simulink model "prach_shortFormat_fftShift_chanfix"  (R2022a)
settings: Solver=FixedStepDiscrete  StartTime=0.0  StopTime=prach_short.SimulationTime  FixedStep=1  RelTol=1e-3  EnableMultiTasking=on
PreLoadFcn:
  | warning off Simulink:Commands:SetParamLinkChangeWarn
  | warning off Simulink:Commands:LoadMdlParameterizedLink
  | warning off Simulink:SL_SetParamLinkChangeWarn
  | warning off Simulink:SL_LoadMdlParameterizedLink
  | setup_prach_shortFormat_fftShift;
InitFcn:
  | setup_prach_shortFormat_fftShift;
StopFcn:
  | figure;
  | subplot(3,1,1);
  | plot(real(X(:,1))/max(real(X(:,1))),'b');
  | hold on;
  | plot(imag(X(:,1))/max(real(X(:,1))),'r');
  | title('Raw FFT output, matlab reference');
  | subplot(3,1,2);
  | plot(real(PrachOut_DSPBA(1:Nfft))/max(real(PrachOut_DSPBA(1:Nfft))), 'k');
  | hold on;
  | plot(imag(PrachOut_DSPBA(1:Nfft))/max(imag(PrachOut_DSPBA(1:Nfft))), 'm');
  | title('Raw FFT output, DSP Builder');
  | subplot(3,1,3);
  | plot(real(X(:,1))/max(real(X(:,1)))-real(PrachOut_DSPBA(1:Nfft))/max(real(PrachOut_DSPBA(1:Nfft))), 'g');
  | hold on;
  | plot(imag(X(:,1))/max(real(X(:,1)))-imag(PrachOut_DSPBA(1:Nfft))/max(imag(PrachOut_DSPBA(1:Nfft))), 'c');
  | title('Difference');
  | 
  | figure;
  | subplot(2,1,1);
  | plot(real(prach_output(:,1))/max(real(prach_output(:,1))),'b');
  | hold on;
  | plot(imag(prach_output(:,1))/max(real(prach_output(:,1))),'r');
  | title('PRACH output, matlab, normalized ');
  | subplot(2,1,2);
  | for i=1:139
  |     PrachOut139reordered_DSPBA(1+PrachIdxOut139_DSPBA(i)) = PrachOut139_DSPBA(i);
  | end;
  | plot(real(PrachOut139reordered_DSPBA)/max(real(PrachOut139reordered_DSPBA)), 'k');
  | hold on;
  | plot(imag(PrachOut139reordered_DSPBA)/max(imag(PrachOut139reordered_DSPBA)), 'm');
  | title('PRACH output, DSP Builder, normalized');
values from neighbouring files (symbols this model uses):
  ConfigTable = [16 1 9,20,20,20,20,20,20,20,20,20 0 2 6 2 4 ... (first row only)    [ConfigIndexTable.m]
  NTxAnts = 4    [setup_prach_shortFormat.m]    (also in setup_prach_shortFormat_fftShift.m)
undefined symbols (not defined in the file or in its folder): AdvDSPBChannelOutDisplay, AdvDSPBDMemDisplay, BW, ControlDecode, display, dpoly, dspba, dspba_ChannelInVis, dspba_ChannelOutVis, dspba_internal_get_channel_ports, evalAionMaskParam, latency, PRACH_CC, PRACH_regs, prach_short, PrachLib, PrachLib_FFTshift, primtype, RemoveCP, Stream2BlockConv, UseDontCare, value, waveconfig
libraries: DSPBAPrim x326, DSPBAControl x10, DSPBAModelBus x7, DSPBABase x5, DSPBAUtilities x5, simulink x2, DSPBAVectorUtil x1, DspbAdvFftLibrary x1
(part 1 of 5)
Description:
  | This design Implements a PRACH detection for short format for TDD configurations.
settings Model: Creator=lrigby  LastModifiedBy=5g
settings SolverCC: AlgebraicLoopSolver=TrustRegion
settings DataIOCC: LimitDataPoints=on  SaveFormat=StructureWithTime  SignalLoggingSaveFormat=ModelDataLogs  ReturnWorkspaceOutputs=off
settings OptimizationCC: ExpressionDepthLimit=2147483647  InitFltsAndDblsToZero=on  LifeSpan=inf
settings DebuggingCC: SaveWithParameterizedLinksMsg=none  UnderspecifiedInitializationDetection=Classic  MergeDetectMultiDrivingBlocksExec=none  SignalResolutionControl=TryResolveAllWithWarning  SolverPrmCheckMsg=warning  ParameterPrecisionLossMsg=none  UnconnectedInputMsg=warning  UnconnectedOutputMsg=warning  UnconnectedLineMsg=warning  StateNameClashWarn=warning  SFUnexpectedBacktrackingDiag=warning  SFNoUnconditionalDefaultTransitionDiag=warning  SFExecutionAtInitializationDiag=none  ArithmeticOperatorsInVariantConditions=warning
settings HardwareCC: ProdBitPerPointer=32  ProdBitPerSizeT=32  ProdBitPerPtrDiffT=32  ProdLargestAtomicFloat=None  ProdIntDivRoundTo=Undefined  ProdEndianess=Unspecified  ProdWordSize=32  ProdHWDeviceType=ASIC/FPGA  TargetBitPerLong=64  TargetBitPerPointer=64  TargetBitPerSizeT=64  TargetBitPerPtrDiffT=64  TargetLongLongMode=on  TargetIntDivRoundTo=Zero  TargetEndianess=LittleEndian  TargetWordSize=64  TargetHWDeviceType=MATLAB Host  ProdEqTarget=off
settings ModelReferenceCC: PropagateSignalLabelsOutOfModel=off
settings SFSimCC: SimUseLocalCustomCode=off  SimParseCustomCode=off  CustomCodeUndefinedFunction=UseInterfaceOnly
settings RTWCC: RTWUseLocalCustomCode=off  DLArmComputeVersion=19.05
settings CodeAppCC: StateflowObjectComments=on
settings GRTTargetCC: TargetFcnLib=ansi_tfl_tmw.mat  TargetLangStandard=C89/C90 (ANSI)  CombineOutputUpdateFcns=off  GRTInterface=on
settings ConfigComp: CovMetricSettings=dw  CovSaveCumulativeToWorkspaceVar=on  CovSaveSingleToWorkspaceVar=on  CovExternalEMLEnable=off  CovSFcnEnable=off

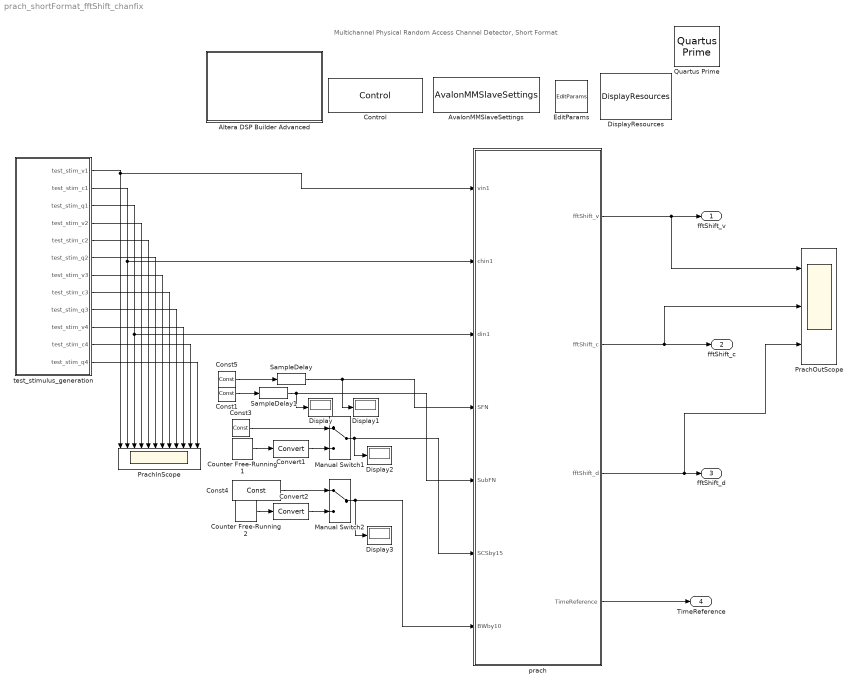
== system prach_shortFormat_fftShift_chanfix ==
  note: Multichannel Physical Random
      | Access Channel Detector, Short Format
  Altera DSP Builder Advanced : Subsystem  mask(DSP Builder Advanced Blockset Ignored Block){}
      settings: OpenFcn=web('http://www.altera.com', '-new');
      mask Display: image(imread('alteralogo.tif'));
  AvalonMMSlaveSettings : DSPBABase/AvalonMMSlaveSettings
  Const1 : DSPBAPrim/Const  primtype=const  nInputs=0  nOutputs=1  omode=Specify via dialog  otype=uint(8)  scale=2^-0  rndmethod=Unbiased  factor=1  satmethod=Symmetric  shift_vec=[0 1 2 -1]  value=SubF  inPortNames=['+'; '+';]  outPortNames=[' ']  dspbaimage=dspba_prim.svg  text=fprintf('%s', num2str(value));  style=Optimised  visibilities=8 + 1024  floatPrecision=float32_m23  warnSaturation=on  version=20211007  SampleTime=inf
  Const3 : DSPBAPrim/Const  primtype=const  nInputs=0  nOutputs=1  omode=Specify via dialog  otype=uint(2)  scale=1  rndmethod=Unbiased  factor=1  satmethod=Symmetric  shift_vec=[0 1 2 -1]  value=floor(waveconfig.PRACH.Config.SubcarrierSpacing/15)  inPortNames=['+'; '+';]  outPortNames=[' ']  dspbaimage=dspba_prim.svg  text=fprintf('%s', num2str(value));  style=Optimised  visibilities=8 + 1024  floatPrecision=float32_m23  warnSaturation=on  version=20211007  SampleTime=inf
  Const4 : DSPBAPrim/Const  primtype=const  nInputs=0  nOutputs=1  omode=Specify via dialog  otype=uint(4)  scale=1  rndmethod=Unbiased  factor=1  satmethod=Symmetric  shift_vec=[0 1 2 -1]  value=floor(BW/10)  inPortNames=['+'; '+';]  outPortNames=[' ']  dspbaimage=dspba_prim.svg  text=fprintf('%s', num2str(value));  style=Optimised  visibilities=8 + 1024  floatPrecision=float32_m23  warnSaturation=on  version=20211007  SampleTime=inf
  Const5 : DSPBAPrim/Const  primtype=const  nInputs=0  nOutputs=1  omode=Specify via dialog  otype=uint(12)  scale=2^-0  rndmethod=Unbiased  factor=1  satmethod=Symmetric  shift_vec=[0 1 2 -1]  value=SFN  inPortNames=['+'; '+';]  outPortNames=[' ']  dspbaimage=dspba_prim.svg  text=fprintf('%s', num2str(value));  style=Optimised  visibilities=8 + 1024  floatPrecision=float32_m23  warnSaturation=on  version=20211007  SampleTime=inf
  Control : DSPBABase/Control  generate=on  language=VHDL  destination=./rtl  make_full_path=off  path_is_relative=on  autotestbench=on  signaldepth=2  coveragetestbench=off  logs=off  spacewidth=2  spacenum=1  addrwidth=10  datawidth=16  dataendian=Big Endian  hierarchicalnames=on  ramThresholdBits=-1  distRamThresholdBits=-1  mlabThresholdBits=-1  hardMultiplierThresholdLuts=-1  version=20090407  errorOnChanMismatch=1  errorOnGPIOMismatch=0  importModelsimResults=0  cycleAccurate=off  reinterpretCastMult=off  paramFile=prach_shortFormat_fftShift_params.xml
  Convert1 : DSPBAPrim/Convert  primtype=convert  nInputs=1  nOutputs=1  omode=Specify via dialog  otype=uint(2)  scale=1  rndmethod=Biased  factor=1  satmethod=None  shift_vec=[0 1 2 -1]  value=round([0:255]/17)  inPortNames=[' '; ' ';]  outPortNames=[' '; 'c']  dspbaimage=dspba_prim_wide.svg  text=fprintf('convert');  style=Optimised  visibilities=8+64+256+2^17  clipdetect=off  floatPrecision=float32_m23  advOptions=[]  version=20211007
  Convert2 : DSPBAPrim/Convert  primtype=convert  nInputs=1  nOutputs=1  omode=Specify via dialog  otype=uint(8)  scale=1  rndmethod=Biased  factor=1  satmethod=None  shift_vec=[0 1 2 -1]  value=round([0:255]/17)  inPortNames=[' '; ' ';]  outPortNames=[' '; 'c']  dspbaimage=dspba_prim_wide.svg  text=fprintf('convert');  style=Optimised  visibilities=8+64+256+2^17  clipdetect=off  floatPrecision=float32_m23  advOptions=[]  version=20211007
  Counter Free-Running1 : simulink/Sources/Counter Free-Running  NumBits=2  tsamp=-1
  Counter Free-Running2 : simulink/Sources/Counter Free-Running  NumBits=4  tsamp=-1
  Display{,1..3} (4 alike) : Display
  DisplayResources : DSPBAUtilities/DisplayResources  mults=0  luts=0  memorybits=0
  EditParams : DSPBABase/EditParams  version=20090407
  Manual Switch1 : ManualSwitch
  Manual Switch2 : ManualSwitch
  PrachInScope : Scope  NumInputPorts=12
  PrachOutScope : Scope  NumInputPorts=3
  Quartus Prime : DSPBABase/Quartus Prime  version=20090407
  SampleDelay : DSPBAPrim/SampleDelay  primtype=sampdelay  nInputs=1  nOutputs=1  omode=Inherit via internal rule  otype=sfix(16)  scale=2^-15  rndmethod=Unbiased  factor=1  satmethod=Symmetric  shift_vec=[0 1 2 -1]  floatPrecision=float32_m23  value=0  inPortNames=[' '; ' ';]  outPortNames=[' ']  dspbaimage=dspba_prim.svg  text=dpoly(1, eye(1,value+1), 'z')  style=Optimised  visibilities=8 + 1024 + 2^17 + 2^18  flexible=off  slackgroup=0  augmented=0  version=20211007  advOptions=[]
  SampleDelay1 : DSPBAPrim/SampleDelay  primtype=sampdelay  nInputs=1  nOutputs=1  omode=Inherit via internal rule  otype=sfix(16)  scale=2^-15  rndmethod=Unbiased  factor=1  satmethod=Symmetric  shift_vec=[0 1 2 -1]  floatPrecision=float32_m23  value=0  inPortNames=[' '; ' ';]  outPortNames=[' ']  dspbaimage=dspba_prim.svg  text=dpoly(1, eye(1,value+1), 'z')  style=Optimised  visibilities=8 + 1024 + 2^17 + 2^18  flexible=off  slackgroup=0  augmented=0  version=20211007  advOptions=[]
  prach : Subsystem
  test_stimulus_generation : Subsystem
  fftShift_v : Outport
  fftShift_c : Outport  Port=2
  fftShift_d : Outport  Port=3
  TimeReference : Outport  Port=4
  wires:
  test_stimulus_generation/2(test_stim_c1) -> PrachInScope/2, prach/2(chin1)
  test_stimulus_generation/3(test_stim_q1) -> PrachInScope/3, prach/3(din1)
  test_stimulus_generation/4(test_stim_v2) -> PrachInScope/4
  test_stimulus_generation/5(test_stim_c2) -> PrachInScope/5
  test_stimulus_generation/6(test_stim_q2) -> PrachInScope/6
  test_stimulus_generation/7(test_stim_v3) -> PrachInScope/7
  test_stimulus_generation/8(test_stim_c3) -> PrachInScope/8
  test_stimulus_generation/9(test_stim_q3) -> PrachInScope/9
  test_stimulus_generation/10(test_stim_v4) -> PrachInScope/10
  test_stimulus_generation/11(test_stim_c4) -> PrachInScope/11
  test_stimulus_generation/12(test_stim_q4) -> PrachInScope/12
  test_stimulus_generation/1(test_stim_v1) -> PrachInScope/1, prach/1(vin1)
  Const5/1 -> SampleDelay/1
  Const1/1 -> SampleDelay1/1
  Const3/1 -> Manual Switch1/1
  Const4/1 -> Manual Switch2/1
  Manual Switch1/1 -> prach/6(SCSby15), Display2/1
  Manual Switch2/1 -> prach/7(BWby10), Display3/1
  Counter Free-Running1/1 -> Convert1/1
  Convert1/1 -> Manual Switch1/2
  Counter Free-Running2/1 -> Convert2/1
  Convert2/1 -> Manual Switch2/2
  SampleDelay/1 -> Display1/1, prach/4(SFN)
  SampleDelay1/1 -> Display/1, prach/5(SubFN)
  prach/2(fftShift_c) -> PrachOutScope/2, fftShift_c/1
  prach/4(TimeReference) -> TimeReference/1
  prach/1(fftShift_v) -> PrachOutScope/1, fftShift_v/1
  prach/3(fftShift_d) -> PrachOutScope/3, fftShift_d/1

== system prach_shortFormat_fftShift_chanfix/Altera DSP Builder Advanced ==

== system prach_shortFormat_fftShift_chanfix/prach ==
  vin1 : Inport
  chin1 : Inport  Port=2
  din1 : Inport  Port=3
  SFN : Inport  Port=4
  SubFN : Inport  Port=5
  SCSby15 : Inport  Port=6
  BWby10 : Inport  Port=7
  Device : DSPBABase/Device  family=Stratix IV  deviceMember=Stratix IV E  stratix4device=Stratix IV E  hardcopy4device=HardCopy IV E  stratix5device=Stratix V GX  device=AUTO  speed=-3  stratixSpeed=-5  stratix2Speed=-3  stratix3Speed=-3  stratix4gxSpeed=-2  stratix4gtSpeed=-1  cyclone2Speed=-6  cyclone3Speed=-6  arria2Speed=-4  cyclone4eSpeed=-8  stratix5Speed=-3  arria5Speed=-4  arriaSpeed=-6  cyclone3lsSpeed=-7  cyclone5Speed=-6  arria2gzSpeed=-3  nightFurySpeed=-2  ecp2Speed=-7  hardcopycompat=off  version=20140217  max10flashmode=off  max10nomeminit=off
  PRACH_CC : Subsystem  AncestorBlock=PrachLib_FFTshift/PRACH_CC  mask{InstanceNumber=1}
      mask prompts: InstanceNumber "CC Index"
      mask init:
      | InstanceNumberStr = num2str(InstanceNumber)
      mask Display:
      | color('w');image('dspba_prim.jpg');
      | fprintf('Component\nCarrier\n\n %s\n\nPRACH', int2str(InstanceNumber));
      | port_label('input',1,'din');
      | port_label('input',2,'vin');
      | port_label('input',3,'chin');
      | port_label('input',4,'SFN');
      | port_label('input',5,'SubFN');
      | port_label('input',6,'SCS/15');
      | port_label('input',7,'BW/10');
      | port_label('output',1,'qv');
      | port_label('output',2,'qc');
      | port_label('output',3,'q');
      | port_label('output',4,'qv139');
      | port_label('output',5,'qFFTBinIdx');
  Scope : Scope  NumInputPorts=4
  Scope1 : Scope  NumInputPorts=4
  Scope2 : Scope  NumInputPorts=4
  log_occupied_bins : Subsystem  TreatAsAtomicUnit=on
  log_occupied_bins1 : Subsystem  TreatAsAtomicUnit=on
  log_raw_fftout : Subsystem  TreatAsAtomicUnit=on
  fftShift_v : Outport
  fftShift_c : Outport  Port=2
  fftShift_d : Outport  Port=3
  TimeReference : Outport  Port=4
  wires:
  vin1/1 -> PRACH_CC/2(vin0)
  chin1/1 -> PRACH_CC/3(chin0)
  SFN/1 -> PRACH_CC/4(SFN)
  SubFN/1 -> PRACH_CC/5(SubFN)
  din1/1 -> PRACH_CC/1(din0)
  SCSby15/1 -> PRACH_CC/6(SCSby15)
  BWby10/1 -> PRACH_CC/7(BWby10)
  PRACH_CC/1(qv) -> log_raw_fftout/Enable, Scope/1
  PRACH_CC/2(qch) -> Scope1/3, log_occupied_bins/2(chin), log_raw_fftout/2(chin), Scope/3
  PRACH_CC/3(q) -> log_occupied_bins/1(din), Scope1/2, Scope/2, log_raw_fftout/1(din)
  PRACH_CC/5(qFreqBinIdx) -> log_occupied_bins/3(FreqBinIdx), Scope1/4, log_raw_fftout/3(FreqBinIdx), Scope/4
  PRACH_CC/4(qv139) -> log_occupied_bins/Enable, Scope1/1
  PRACH_CC/8(fftShift_d) -> fftShift_d/1, log_occupied_bins1/1(din), Scope2/3
  PRACH_CC/9(TimeReference) -> TimeReference/1, Scope2/4
  PRACH_CC/6(fftShift_v) -> fftShift_v/1, Scope2/1, log_occupied_bins1/Enable
  PRACH_CC/7(fftShift_c) -> fftShift_c/1, log_occupied_bins1/2(chin), Scope2/2

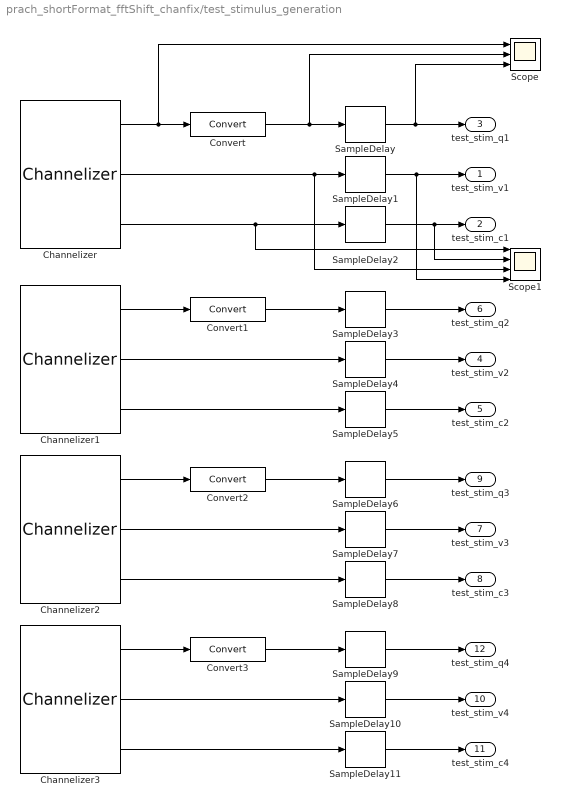
== system prach_shortFormat_fftShift_chanfix/test_stimulus_generation ==
  Channelizer : DSPBAUtilities/Channelizer  data_input=prach_short.din  folding=prach_short.ClockRate/prach_short.SampleRateMSPS  samples_valid=NTxAnts  samples_idle=0  sample_time=prach_short.SampleTime
  Channelizer1 : DSPBAUtilities/Channelizer  data_input=-prach_short.din  folding=prach_short.ClockRate/prach_short.SampleRateMSPS  samples_valid=NTxAnts  samples_idle=1  sample_time=prach_short.SampleTime
  Channelizer2 : DSPBAUtilities/Channelizer  data_input=prach_short.din  folding=prach_short.ClockRate/prach_short.SampleRateMSPS  samples_valid=NTxAnts  samples_idle=2  sample_time=prach_short.SampleTime
  Channelizer3 : DSPBAUtilities/Channelizer  data_input=-prach_short.din  folding=prach_short.ClockRate/prach_short.SampleRateMSPS  samples_valid=NTxAnts  samples_idle=3  sample_time=prach_short.SampleTime
  Convert{,1..3} (4 alike) : DSPBAPrim/Convert  primtype=convert  nInputs=1  nOutputs=1  omode=Specify via dialog  otype=sfix(16)  scale=2^-15  rndmethod=Biased  factor=1  satmethod=None  shift_vec=[0 1 2 -1]  value=round([0:255]/17)  inPortNames=[' '; ' ';]  outPortNames=[' '; 'c']  dspbaimage=dspba_prim_wide.svg  text=fprintf('convert');  style=Optimised  visibilities=8+64+256+2^17  clipdetect=off  floatPrecision=float32_m23  advOptions=[]  version=20211007
  SampleDelay{,1..6,8..9,11} (10 alike) : DSPBAPrim/SampleDelay  primtype=sampdelay  nInputs=1  nOutputs=1  omode=Inherit via internal rule  otype=sfix(16)  scale=2^-15  rndmethod=Unbiased  factor=1  satmethod=Symmetric  shift_vec=[0 1 2 -1]  floatPrecision=float32_m23  value=0  inPortNames=[' '; ' ';]  outPortNames=[' ']  dspbaimage=dspba_prim.svg  text=dpoly(1, eye(1,value+1), 'z')  style=Optimised  visibilities=8 + 1024 + 2^17 + 2^18  flexible=off  slackgroup=0  augmented=0  version=20211007  advOptions=[]
  SampleDelay10 : DSPBAPrim/SampleDelay  primtype=sampdelay  nInputs=1  nOutputs=1  omode=boolean  otype=sfix(16)  scale=2^-15  rndmethod=Unbiased  factor=1  satmethod=Symmetric  shift_vec=[0 1 2 -1]  floatPrecision=float32_m23  value=0  inPortNames=[' '; ' ';]  outPortNames=[' ']  dspbaimage=dspba_prim.svg  text=dpoly(1, eye(1,value+1), 'z')  style=Optimised  visibilities=8 + 1024 + 2^17 + 2^18  flexible=off  slackgroup=0  augmented=0  version=20211007  advOptions=[]
  SampleDelay7 : DSPBAPrim/SampleDelay  primtype=sampdelay  nInputs=1  nOutputs=1  omode=boolean  otype=sfix(16)  scale=2^-15  rndmethod=Unbiased  factor=1  satmethod=Symmetric  shift_vec=[0 1 2 -1]  floatPrecision=float32_m23  value=0  inPortNames=[' '; ' ';]  outPortNames=[' ']  dspbaimage=dspba_prim.svg  text=dpoly(1, eye(1,value+1), 'z')  style=Optimised  visibilities=8 + 1024 + 2^17 + 2^18  flexible=off  slackgroup=0  augmented=0  version=20211007  advOptions=[]
  Scope : Scope  NumInputPorts=3
  Scope1 : Scope  NumInputPorts=4
  test_stim_v1 : Outport  VectorParamsAs1DForOutWhenUnconnected=off
  test_stim_c1 : Outport  Port=2  VectorParamsAs1DForOutWhenUnconnected=off
  test_stim_q1 : Outport  Port=3  VectorParamsAs1DForOutWhenUnconnected=off
  test_stim_v2 : Outport  Port=4  VectorParamsAs1DForOutWhenUnconnected=off
  test_stim_c2 : Outport  Port=5  VectorParamsAs1DForOutWhenUnconnected=off
  test_stim_q2 : Outport  Port=6  VectorParamsAs1DForOutWhenUnconnected=off
  test_stim_v3 : Outport  Port=7  VectorParamsAs1DForOutWhenUnconnected=off
  test_stim_c3 : Outport  Port=8  VectorParamsAs1DForOutWhenUnconnected=off
  test_stim_q3 : Outport  Port=9  VectorParamsAs1DForOutWhenUnconnected=off
  test_stim_v4 : Outport  Port=10  VectorParamsAs1DForOutWhenUnconnected=off
  test_stim_c4 : Outport  Port=11  VectorParamsAs1DForOutWhenUnconnected=off
  test_stim_q4 : Outport  Port=12  VectorParamsAs1DForOutWhenUnconnected=off
  wires:
  Channelizer/1 -> Scope/1, Convert/1
  Convert/1 -> Scope/2, SampleDelay/1
  SampleDelay/1 -> Scope/3, test_stim_q1/1
  SampleDelay2/1 -> Scope1/2, test_stim_c1/1
  Channelizer/2 -> Scope1/3, SampleDelay1/1
  SampleDelay5/1 -> test_stim_c2/1
  SampleDelay3/1 -> test_stim_q2/1
  Channelizer1/3 -> SampleDelay5/1
  Channelizer1/2 -> SampleDelay4/1
  Convert1/1 -> SampleDelay3/1
  Channelizer1/1 -> Convert1/1
  SampleDelay8/1 -> test_stim_c3/1
  SampleDelay6/1 -> test_stim_q3/1
  Channelizer2/3 -> SampleDelay8/1
  Channelizer2/2 -> SampleDelay7/1
  Convert2/1 -> SampleDelay6/1
  Channelizer2/1 -> Convert2/1
  Channelizer3/2 -> SampleDelay10/1
  SampleDelay9/1 -> test_stim_q4/1
  Convert3/1 -> SampleDelay9/1
  Channelizer3/1 -> Convert3/1
  Channelizer3/3 -> SampleDelay11/1
  SampleDelay11/1 -> test_stim_c4/1
  SampleDelay4/1 -> test_stim_v2/1
  SampleDelay1/1 -> Scope1/4, test_stim_v1/1
  Channelizer/3 -> Scope1/1, SampleDelay2/1
  SampleDelay7/1 -> test_stim_v3/1
  SampleDelay10/1 -> test_stim_v4/1

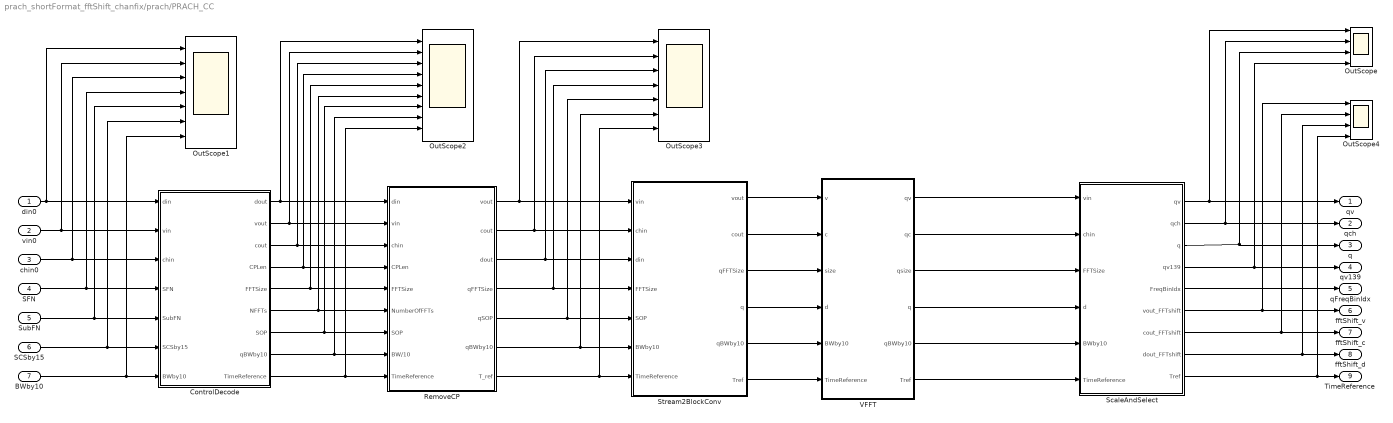
== system prach_shortFormat_fftShift_chanfix/prach/PRACH_CC ==
  din0 : Inport
  vin0 : Inport  Port=2
  chin0 : Inport  Port=3
  SFN : Inport  Port=4
  SubFN : Inport  Port=5
  SCSby15 : Inport  Port=6
  BWby10 : Inport  Port=7
  ControlDecode : Subsystem  AncestorBlock=PrachLib/ControlDecode  mask{InstanceNumber=InstanceNumber}
      mask prompts: InstanceNumber "CC Index"
  OutScope : Scope  NumInputPorts=4
  OutScope1 : Scope  NumInputPorts=7
  OutScope2 : Scope  NumInputPorts=9
  OutScope3 : Scope  NumInputPorts=7
  OutScope4 : Scope  NumInputPorts=4
  RemoveCP : Subsystem  AncestorBlock=PrachLib/RemoveCP  mask{NAnts=NTxAnts}
      mask prompts: NAnts "Number of Antennas"
  ScaleAndSelect : Subsystem
  Stream2BlockConv : Subsystem  AncestorBlock=PrachLib/Stream2BlockConv  mask{NAnts=4, NFftMax=prach_short.Nfft}
      mask prompts: NAnts "Number of Antennas"; NFftMax "Maximum FFT size"
  VFFT : Subsystem  AncestorBlock=DspbAdvFftLibrary/Common/VFFT  Opaque=on  mask{IFFT=false, subchannels=1, br_in=true, maxSize=log2(prach_short.Nfft), minSize=9, in_type=prach_short.InputType, type_strings=prach_short.type_strings, faithful=false}
      mask prompts: subchannels "Number of interleaved subchannels (must be a power of 2)"; br_in "Bit-reversed input"; maxSize "maxSize, where the (I)FFT has at most 2^maxSize points"; minSize "minSize, where the (I)FFT has at least 2^minSize points"; in_type "Input type"; type_strings "Twiddle/pruning specification"; faithful "Use faithful rounding"
      mask init:
      | block = gcb;
      | 
      | % Check that we have a legal number of subchannels
      | subchannelbits = ceil(log2(subchannels));
      | if not(subchannels == 2^subchannelbits)
      |     error('%s: subchannels count %d is not a power of 2', block, subchannels);
      | end
      | 
      | if IFFT
      |     FFTstring = 'IFFT';
      | else
      |     FFTstring = 'FFT';
      | end
      | 
      | if br_in
      |     directionString = 'BR->NAT';
      | else
      |     directionString = 'NAT->BR';
      | end
      | 
      | if 1 < subchannels
      |     subchannelString = sprintf('%d subchannels',subchannels);
      | else
      |     subchannelString = '';
      | end
      mask Help: helpview(dspba.GetHelp('fft'));
      mask Display:
      | color('w');
      | image('dspba_fft.jpg');
      | port_label('input',1,'v');
      | port_label('input',2,'c');
      | port_label('input',3,'size');
      | port_label('input',4,'d');
      | port_label('input',5,'BW/10');
      | port_label('output',1,'qv');
      | port_label('output',2,'qc');
      | port_label('output',3,'qsize');
      | port_label('output',4,'q');
      | port_label('output',5,'qBW/10');
      | text(0.30,0.65,sprintf('V%s Core',FFTstring));
      | text(0.35,0.55,sprintf('2^{%d} to 2^{%d}',minSize,maxSize),'texmode','on');
      | text(0.30,0.45,directionString);
      | text(0.20,0.30,subchannelString);
  qv : Outport
  qch : Outport  Port=2
  q : Outport  Port=3
  qv139 : Outport  Port=4
  qFreqBinIdx : Outport  Port=5
  fftShift_v : Outport  Port=6
  fftShift_c : Outport  Port=7
  fftShift_d : Outport  Port=8
  TimeReference : Outport  Port=9
  wires:
  ControlDecode/8(qBWby10) -> OutScope2/8, RemoveCP/8(BW/10)
  ControlDecode/7(SOP) -> OutScope2/7, RemoveCP/7(SOP)
  ControlDecode/6(NFFTs) -> OutScope2/6, RemoveCP/6(NumberOfFFTs)
  ControlDecode/5(FFTSize) -> OutScope2/5, RemoveCP/5(FFTSize)
  ControlDecode/4(CPLen) -> OutScope2/4, RemoveCP/4(CPLen)
  ControlDecode/3(cout) -> OutScope2/3, RemoveCP/3(chin)
  ControlDecode/2(vout) -> OutScope2/2, RemoveCP/2(vin)
  ControlDecode/1(dout) -> OutScope2/1, RemoveCP/1(din)
  Stream2BlockConv/4(q) -> VFFT/4(d)
  Stream2BlockConv/3(qFFTSize) -> VFFT/3(size)
  Stream2BlockConv/2(cout) -> VFFT/2(c)
  Stream2BlockConv/1(vout) -> VFFT/1(v)
  VFFT/5(qBWby10) -> ScaleAndSelect/5(BWby10)
  Stream2BlockConv/5(qBWby10) -> VFFT/5(BWby10)
  ScaleAndSelect/5(FreqBinIdx) -> qFreqBinIdx/1
  ScaleAndSelect/3(q) -> OutScope/3, q/1
  ScaleAndSelect/2(qch) -> OutScope/2, qch/1
  ScaleAndSelect/1(qv) -> OutScope/1, qv/1
  VFFT/4(q) -> ScaleAndSelect/4(d)
  VFFT/3(qsize) -> ScaleAndSelect/3(FFTSize)
  VFFT/2(qc) -> ScaleAndSelect/2(chin)
  VFFT/1(qv) -> ScaleAndSelect/1(vin)
  SCSby15/1 -> OutScope1/6, ControlDecode/6(SCSby15)
  vin0/1 -> OutScope1/2, ControlDecode/2(vin)
  chin0/1 -> OutScope1/3, ControlDecode/3(chin)
  SubFN/1 -> OutScope1/5, ControlDecode/5(SubFN)
  din0/1 -> OutScope1/1, ControlDecode/1(din)
  SFN/1 -> OutScope1/4, ControlDecode/4(SFN)
  ScaleAndSelect/7(cout_FFTshift) -> OutScope4/2, fftShift_c/1
  ScaleAndSelect/6(vout_FFTshift) -> OutScope4/1, fftShift_v/1
  ControlDecode/9(TimeReference) -> OutScope2/9, RemoveCP/9(TimeReference)
  Stream2BlockConv/6(Tref) -> VFFT/6(TimeReference)
  VFFT/6(Tref) -> ScaleAndSelect/6(TimeReference)
  ScaleAndSelect/9(Tref) -> OutScope4/4, TimeReference/1
  ScaleAndSelect/4(qv139) -> qv139/1, OutScope/4
  BWby10/1 -> OutScope1/7, ControlDecode/7(BWby10)
  RemoveCP/3(dout) -> OutScope3/3, Stream2BlockConv/3(din)
  RemoveCP/6(qBWby10) -> OutScope3/6, Stream2BlockConv/6(BWby10)
  RemoveCP/1(vout) -> OutScope3/1, Stream2BlockConv/1(vin)
  RemoveCP/4(qFFTSize) -> OutScope3/4, Stream2BlockConv/4(FFTSize)
  RemoveCP/2(cout) -> OutScope3/2, Stream2BlockConv/2(chin)
  RemoveCP/7(T_ref) -> OutScope3/7, Stream2BlockConv/7(TimeReference)
  RemoveCP/5(qSOP) -> OutScope3/5, Stream2BlockConv/5(SOP)
  ScaleAndSelect/8(dout_FFTshift) -> OutScope4/3, fftShift_d/1

== system prach_shortFormat_fftShift_chanfix/prach/log_occupied_bins ==
  din : Inport
  chin : Inport  Port=2
  FreqBinIdx : Inport  Port=3
  Enable : EnablePort
  To Workspace : ToWorkspace  VariableName=PrachOut139_DSPBA  SampleTime=-1
  To Workspace1 : ToWorkspace  VariableName=PrachIdxOut139_DSPBA  SampleTime=-1
  To Workspace2 : ToWorkspace  VariableName=PrachAntOut139_DSPBA  SampleTime=-1
  wires:
  chin/1 -> To Workspace2/1
  din/1 -> To Workspace/1
  FreqBinIdx/1 -> To Workspace1/1

== system prach_shortFormat_fftShift_chanfix/prach/log_occupied_bins1 ==
  din : Inport
  chin : Inport  Port=2
  Enable : EnablePort
  To Workspace : ToWorkspace  VariableName=PrachOut139_fftShift  SampleTime=-1
      settings: Save2DSignal=2-D array (concatenate along first dimension)
  To Workspace2 : ToWorkspace  VariableName=PrachAntOut139_fftShift  SampleTime=-1
  wires:
  din/1 -> To Workspace/1
  chin/1 -> To Workspace2/1

== system prach_shortFormat_fftShift_chanfix/prach/log_raw_fftout ==
  din : Inport
  chin : Inport  Port=2
  FreqBinIdx : Inport  Port=3
  Enable : EnablePort
  To Workspace : ToWorkspace  VariableName=PrachOut_DSPBA  SampleTime=-1
  To Workspace1 : ToWorkspace  VariableName=PrachIdxOut_DSPBA  SampleTime=-1
  To Workspace2 : ToWorkspace  VariableName=PrachAntOut_DSPBA  SampleTime=-1
  wires:
  FreqBinIdx/1 -> To Workspace1/1
  din/1 -> To Workspace/1
  chin/1 -> To Workspace2/1

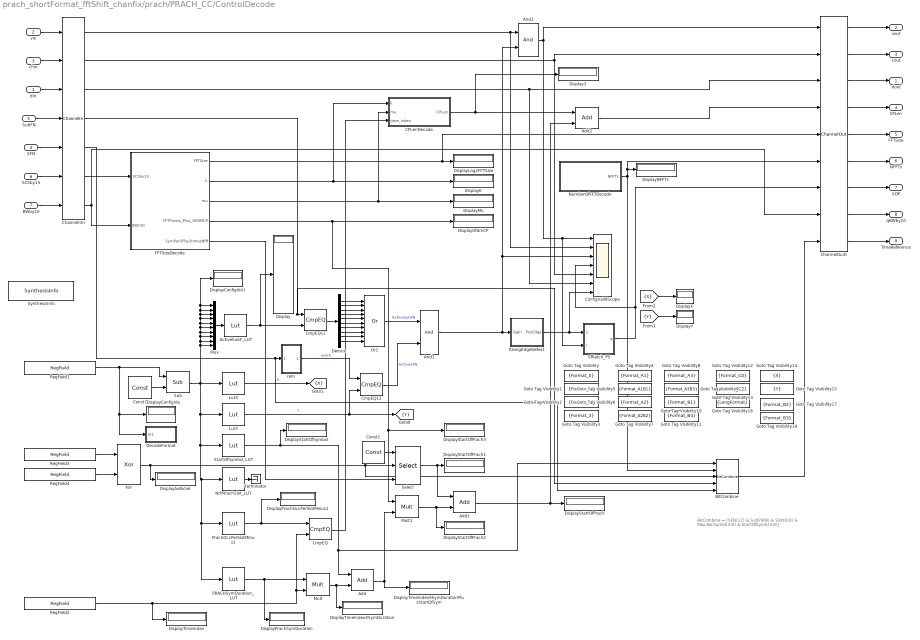
== system prach_shortFormat_fftShift_chanfix/prach/PRACH_CC/ControlDecode ==
  note: BitCombine = [SFN(12) & SubFN(8) & SlotID(0) & Max.No.Symbl(3:0) & StartOfSymb(3:0)]
  din : Inport
  vin : Inport  Port=2
  chin : Inport  Port=3
  SFN : Inport  Port=4
  SubFN : Inport  Port=5
  SCSby15 : Inport  Port=6
  BWby10 : Inport  Port=7
  ActiveSubF_LUT : DSPBAPrim/Lut  primtype=lut  nInputs=1  nOutputs=1  omode=Inherit via internal rule  otype=sfix(16)  scale=2^-15  rndmethod=Unbiased  factor=1  satmethod=Symmetric  shift_vec=[0 1 2 -1]  value=ConfigTable(:,3:12)  inPortNames=[' '; ' ';]  outPortNames=[' ']  dspbaimage=dspba_prim.svg  text=fprintf('LUT');  style=Optimised  visibilities=8 + 1024  floatPrecision=float32_m23  version=20211007
  Add : DSPBAPrim/Add  primtype=add  nInputs=evalAionMaskParam(gcb,'value',1)  nOutputs=1  omode=Inherit via internal rule with word growth  otype=sfix(16)  scale=2^-15  rndmethod=Unbiased  factor=1  satmethod=Symmetric  shift_vec=[0 1 2 -1]  value=2  inPortNames=[' '; ' ';]  outPortNames=[' ']  dspbaimage=dspba_prim.svg  text=fprintf('+');  style=Optimised  visibilities=1032+2^17+2^18+2^19  genFPC=off  floatRounding=correct  advOptions=[]  version=20211007
  Add1 : DSPBAPrim/Add  primtype=add  nInputs=evalAionMaskParam(gcb,'value',1)  nOutputs=1  omode=Inherit via internal rule with word growth  otype=sfix(16)  scale=2^-15  rndmethod=Unbiased  factor=1  satmethod=Symmetric  shift_vec=[0 1 2 -1]  value=2  inPortNames=[' '; ' ';]  outPortNames=[' ']  dspbaimage=dspba_prim.svg  text=fprintf('+');  style=Optimised  visibilities=1032+2^17+2^18+2^19  genFPC=off  floatRounding=correct  advOptions=[]  version=20211007
  Add2 : DSPBAPrim/Add  primtype=add  nInputs=evalAionMaskParam(gcb,'value',1)  nOutputs=1  omode=Inherit via internal rule with word growth  otype=sfix(16)  scale=2^-15  rndmethod=Unbiased  factor=1  satmethod=Symmetric  shift_vec=[0 1 2 -1]  value=2  inPortNames=[' '; ' ';]  outPortNames=[' ']  dspbaimage=dspba_prim.svg  text=fprintf('+');  style=Optimised  visibilities=1032+2^17+2^18+2^19  genFPC=off  floatRounding=correct  advOptions=[]  version=20211007
  And1 : DSPBAPrim/And  primtype=and  nInputs=2  nOutputs=1  omode=Inherit via internal rule  otype=sfix(16)  scale=2^-15  rndmethod=Unbiased  factor=1  satmethod=Symmetric  shift_vec=[0 1 2 -1]  value=0  inPortNames=[' '; ' '; ' '; ' '; ' '; ' '; ' '; ' '; ' '; ' '; ' '; ' '; ' '; ' '; ' '; ' '; ]  outPortNames=[' ']  dspbaimage=dspba_prim.svg  text=fprintf('&');  style=Optimised  visibilities=8+2  version=20211007
  And2 : DSPBAPrim/And  primtype=and  nInputs=2  nOutputs=1  omode=Inherit via internal rule  otype=sfix(16)  scale=2^-15  rndmethod=Unbiased  factor=1  satmethod=Symmetric  shift_vec=[0 1 2 -1]  value=0  inPortNames=[' '; ' '; ' '; ' '; ' '; ' '; ' '; ' '; ' '; ' '; ' '; ' '; ' '; ' '; ' '; ' '; ]  outPortNames=[' ']  dspbaimage=dspba_prim.svg  text=fprintf('&');  style=Optimised  visibilities=8+2  version=20211007
  BitCombine : DSPBAPrim/BitCombine  primtype=bitcombine  nInputs=5  nOutputs=1  omode=Inherit via internal rule  otype=sfix(16)  scale=2^-15  rndmethod=Unbiased  factor=1  satmethod=Symmetric  shift_vec=[0 1 2 -1]  value=0  inPortNames=['l'; 'h';]  outPortNames=[' ']  dspbaimage=dspba_prim.svg  text=fprintf('[h,l]');  style=Optimised  visibilities=8+2  version=20211007
  CPLenDecode : Subsystem
      mask Display:
      | color('w');
      | image('dspba_prim.jpg');
      | port_label('output',1,'CPLen*nAnt');
      | port_label('input',1,'k');
      | port_label('input',2,'mu');
      | port_label('input',3,'time_index');
  ChannelI3n : DSPBAPrim/ChannelIn  primtype=channelin  nInputs=dspba_internal_get_channel_ports(gcb)  nOutputs=dspba_internal_get_channel_ports(gcb)  omode=Inherit via internal rule  otype=sfix(16)  scale=2^-15  rndmethod=Unbiased  factor=1  satmethod=Symmetric  shift_vec=[0 1 2 -1]  value=5  inPortNames=['v'; 'c'; '0'; '1'; '2'; '3'; '4'; '5'; '6'; '7'; '8'; '9'; 'A'; 'B'; 'D'; 'E'; 'F'; 'G'; 'H'; 'I'; 'J'; 'K'; 'L'; 'M'; 'N'; 'O'; 'P'; 'Q'; 'R'; 'S'; 'T'; 'U'; 'W'; 'X'; 'Y'; 'Z']  outPortNames=['v'; 'c'; '0'; '1'; '2'; '3'; '4'; '5'; '6'; '7'; '8'; '9'; 'A'; 'B'; 'D'; 'E'; 'F'; 'G'; 'H'; 'I'; 'J'; 'K'; 'L'; 'M'; 'N'; 'O'; 'P'; 'Q'; 'R'; 'S'; 'T'; 'U'; 'W'; 'X'; 'Y'; 'Z']  dspbaimage=dspba_prim_channel_tall.svg  text=fprintf('In');  style=Optimised  dataSignals=5  foldingEnabled=off  channels=1  sampleRate=200  packetBeginPresent=off  packetBeginEnabled=off  visibilities=dspba_ChannelInVis(gcb)  latencyCorrection=0  scheduleOrigin=off  version=20211214
  ChannelOu3t : DSPBAPrim/ChannelOut  primtype=channelout  nInputs=dspba_internal_get_channel_ports(gcb)  nOutputs=dspba_internal_get_channel_ports(gcb)  omode=Inherit via internal rule  otype=sfix(16)  scale=2^-15  rndmethod=Unbiased  factor=1  satmethod=Symmetric  shift_vec=[0 1 2 -1]  value=7  inPortNames=['v'; 'c'; '0'; '1'; '2'; '3'; '4'; '5'; '6'; '7'; '8'; '9'; 'A'; 'B'; 'D'; 'E'; 'F'; 'G'; 'H'; 'I'; 'J'; 'K'; 'L'; 'M'; 'N'; 'O'; 'P'; 'Q'; 'R'; 'S'; 'T'; 'U'; 'W'; 'X'; 'Y'; 'Z']  outPortNames=['v'; 'c'; '0'; '1'; '2'; '3'; '4'; '5'; '6'; '7'; '8'; '9'; 'A'; 'B'; 'D'; 'E'; 'F'; 'G'; 'H'; 'I'; 'J'; 'K'; 'L'; 'M'; 'N'; 'O'; 'P'; 'Q'; 'R'; 'S'; 'T'; 'U'; 'W'; 'X'; 'Y'; 'Z']  dspbaimage=dspba_prim_channel_tall.svg  text=fprintf('Out%s', AdvDSPBChannelOutDisplay(latency));  style=Optimised  dataSignals=7  foldingEnabled=off  channels=1  sampleRate=200  packetBeginPresent=off  packetBeginEnabled=off  visibilities=dspba_ChannelOutVis(gcb)  latency=14  latencyCorrection=0  version=20211214
  CmpEQ : DSPBAPrim/CmpEQ  primtype=cmpeq  nInputs=2  nOutputs=1  omode=boolean  otype=sfix(16)  scale=2^-15  rndmethod=Unbiased  factor=1  satmethod=Symmetric  shift_vec=[0 1 2 -1]  value=0  inPortNames=[' '; ' ';]  outPortNames=[' ']  dspbaimage=dspba_prim.svg  text=fprintf('==');  style=Optimised  visibilities=0  advOptions=[]  version=20211007
  CmpEQ11 : DSPBAPrim/CmpEQ  primtype=cmpeq  nInputs=2  nOutputs=1  omode=boolean  otype=sfix(16)  scale=2^-15  rndmethod=Unbiased  factor=1  satmethod=Symmetric  shift_vec=[0 1 2 -1]  value=0  inPortNames=[' '; ' ';]  outPortNames=[' ']  dspbaimage=dspba_prim.svg  text=fprintf('==');  style=Optimised  visibilities=0  advOptions=[]  version=20211007
  CmpEQ12 : DSPBAPrim/CmpEQ  primtype=cmpeq  nInputs=2  nOutputs=1  omode=boolean  otype=sfix(16)  scale=2^-15  rndmethod=Unbiased  factor=1  satmethod=Symmetric  shift_vec=[0 1 2 -1]  value=0  inPortNames=[' '; ' ';]  outPortNames=[' ']  dspbaimage=dspba_prim.svg  text=fprintf('==');  style=Optimised  visibilities=0  advOptions=[]  version=20211007
  ConfigValidScope : Scope  NumInputPorts=7
  Const1 : DSPBAPrim/Const  primtype=const  nInputs=0  nOutputs=1  omode=Inherit via internal rule  otype=sfix(16)  scale=2^-15  rndmethod=Unbiased  factor=1  satmethod=Symmetric  shift_vec=[0 1 2 -1]  value=0  inPortNames=['+'; '+';]  outPortNames=[' ']  dspbaimage=dspba_prim.svg  text=fprintf('%s', num2str(value));  style=Optimised  visibilities=8 + 1024  floatPrecision=float32_m23  warnSaturation=on  version=20211007  SampleTime=inf
  Const3 : DSPBAPrim/Const  primtype=const  nInputs=0  nOutputs=1  omode=Inherit via internal rule  otype=sfix(16)  scale=2^-15  rndmethod=Unbiased  factor=1  satmethod=Symmetric  shift_vec=[0 1 2 -1]  value=67  inPortNames=['+'; '+';]  outPortNames=[' ']  dspbaimage=dspba_prim.svg  text=fprintf('%s', num2str(value));  style=Optimised  visibilities=8 + 1024  floatPrecision=float32_m23  warnSaturation=on  version=20211007  SampleTime=inf
  DecodeFormat : Subsystem
  Demux : Demux  Outputs=10
  Display : Display
  Display3 : Display
  DisplayAxBxSel : Display
  DisplayConfigIdx : Display
  DisplayConfigIdx1 : Display
  DisplayK : Display
  DisplayLog2FFTSize : Display
  DisplayMu : Display
  DisplayNFFTs : Display
  DisplayOfdmCP : Display
  DisplayPrachOccPerSlotMinus1 : Display
  DisplayPrachSymDuration : Display
  DisplayStartOfPrach{,1..3} (4 alike) : Display
  DisplayStartOfSymbol : Display
  DisplayTimeIndex : Display
  DisplayTimeIndexXSymDuration : Display
  DisplayTimeIndexXSymDurationPlusStartOfSym : Display
  DisplayX : Display
  DisplayY : Display
  FFTSizeDecode : Subsystem
      mask Display:
      | color('w');
      | image('dspba_prim.jpg');
      | port_label('output',1,'log2(FFT size)');
      | port_label('output',2,'k');
      | port_label('output',3,'mu');
      | port_label('output',4,'FFTPoints+OFDM_CP');
      | port_label('output',5,'SymPerSF/2*Nfft');
      | port_label('input',1,'SCS/15');
      | port_label('input',2,'BW/10');
  Goto Tag Visibility : GotoTagVisibility  GotoTag=Format_0
  Goto Tag Visibility1 : GotoTagVisibility  GotoTag=Format_1
  Goto Tag Visibility10 : GotoTagVisibility  GotoTag=Format_B1
  Goto Tag Visibility11 : GotoTagVisibility  GotoTag=Format_B4
  Goto Tag Visibility12 : GotoTagVisibility  GotoTag=Format_C0
  Goto Tag Visibility13 : GotoTagVisibility  GotoTag=Format_C2
  Goto Tag Visibility14 : GotoTagVisibility  GotoTag=X
  Goto Tag Visibility15 : GotoTagVisibility  GotoTag=Y
  Goto Tag Visibility16 : GotoTagVisibility  GotoTag=LongFormat
  Goto Tag Visibility17 : GotoTagVisibility  GotoTag=Format_B2
  Goto Tag Visibility18 : GotoTagVisibility  GotoTag=Format_B3
  Goto Tag Visibility2 : GotoTagVisibility  GotoTag=Format_2
  Goto Tag Visibility3 : GotoTagVisibility  GotoTag=Format_3
  Goto Tag Visibility4 : GotoTagVisibility  GotoTag=Format_A1
  Goto Tag Visibility5 : GotoTagVisibility  GotoTag=Format_A1B1
  Goto Tag Visibility6 : GotoTagVisibility  GotoTag=Format_A2
  Goto Tag Visibility7 : GotoTagVisibility  GotoTag=Format_A2B2
  Goto Tag Visibility8 : GotoTagVisibility  GotoTag=Format_A3
  Goto Tag Visibility9 : GotoTagVisibility  GotoTag=Format_A3B3
  LutX : DSPBAPrim/Lut  primtype=lut  nInputs=1  nOutputs=1  omode=Inherit via internal rule  otype=sfix(16)  scale=2^-15  rndmethod=Unbiased  factor=1  satmethod=Symmetric  shift_vec=[0 1 2 -1]  value=ConfigTable(:,1)  inPortNames=[' '; ' ';]  outPortNames=[' ']  dspbaimage=dspba_prim.svg  text=fprintf('LUT');  style=Optimised  visibilities=8 + 1024  floatPrecision=float32_m23  version=20211007
  LutY : DSPBAPrim/Lut  primtype=lut  nInputs=1  nOutputs=1  omode=Inherit via internal rule  otype=sfix(16)  scale=2^-15  rndmethod=Unbiased  factor=1  satmethod=Symmetric  shift_vec=[0 1 2 -1]  value=ConfigTable(:,2)  inPortNames=[' '; ' ';]  outPortNames=[' ']  dspbaimage=dspba_prim.svg  text=fprintf('LUT');  style=Optimised  visibilities=8 + 1024  floatPrecision=float32_m23  version=20211007
  Mult : DSPBAPrim/Mult  primtype=mult  nInputs=2  nOutputs=1  omode=Inherit via internal rule  otype=sfix(16)  scale=2^-15  rndmethod=Unbiased  factor=1  satmethod=Symmetric  shift_vec=[0 1 2 -1]  value=0  inPortNames=[' '; ' ';]  outPortNames=[' ']  dspbaimage=dspba_prim.svg  text=fprintf('X');  style=Optimised  visibilities=8+2^18+2^19  floatPrecision=float32_m23  floatRounding=correct  advOptions=[]  version=20211007
  Mult1 : DSPBAPrim/Mult  primtype=mult  nInputs=2  nOutputs=1  omode=Inherit via internal rule  otype=sfix(16)  scale=2^-15  rndmethod=Unbiased  factor=1  satmethod=Symmetric  shift_vec=[0 1 2 -1]  value=0  inPortNames=[' '; ' ';]  outPortNames=[' ']  dspbaimage=dspba_prim.svg  text=fprintf('X');  style=Optimised  visibilities=8+2^18+2^19  floatPrecision=float32_m23  floatRounding=correct  advOptions=[]  version=20211007
  Mux : Mux  Inputs=10
  NrPRrachSlot_LUT : DSPBAPrim/Lut  primtype=lut  nInputs=1  nOutputs=1  omode=Inherit via internal rule  otype=sfix(16)  scale=2^-15  rndmethod=Unbiased  factor=1  satmethod=Symmetric  shift_vec=[0 1 2 -1]  value=ConfigTable(:,14)  inPortNames=[' '; ' ';]  outPortNames=[' ']  dspbaimage=dspba_prim.svg  text=fprintf('LUT');  style=Optimised  visibilities=8 + 1024  floatPrecision=float32_m23  version=20211007
  NumberOfFFTDecode : Subsystem
      mask Display:
      | color('w');
      | image('dspba_prim.jpg');
      | port_label('output',1,'Number of FFTs');
  Or1 : DSPBAPrim/Or  primtype=or  nInputs=10  nOutputs=1  omode=Inherit via internal rule  otype=sfix(16)  scale=2^-15  rndmethod=Unbiased  factor=1  satmethod=Symmetric  shift_vec=[0 1 2 -1]  value=0  inPortNames=[' '; ' '; ' '; ' '; ' '; ' '; ' '; ' '; ' '; ' '; ' '; ' '; ' '; ' '; ' '; ' '; ]  outPortNames=[' ']  dspbaimage=dspba_prim.svg  text=fprintf('|');  style=Optimised  visibilities=8+2  version=20211007
  PRACHSymDuration_LUT : DSPBAPrim/Lut  primtype=lut  nInputs=1  nOutputs=1  omode=Inherit via internal rule  otype=sfix(16)  scale=2^-15  rndmethod=Unbiased  factor=1  satmethod=Symmetric  shift_vec=[0 1 2 -1]  value=ConfigTable(:,16)  inPortNames=[' '; ' ';]  outPortNames=[' ']  dspbaimage=dspba_prim.svg  text=fprintf('LUT');  style=Optimised  visibilities=8 + 1024  floatPrecision=float32_m23  version=20211007
  PrachOccPerSlotMinus1 : DSPBAPrim/Lut  primtype=lut  nInputs=1  nOutputs=1  omode=Inherit via internal rule  otype=sfix(16)  scale=2^-15  rndmethod=Unbiased  factor=1  satmethod=Symmetric  shift_vec=[0 1 2 -1]  value=ConfigTable(:,15)-1  inPortNames=[' '; ' ';]  outPortNames=[' ']  dspbaimage=dspba_prim.svg  text=fprintf('LUT');  style=Optimised  visibilities=8 + 1024  floatPrecision=float32_m23  version=20211007
  RegField1 : DSPBAModelBus/RegField  reg_name=PRACH_regs(InstanceNumber).PRACH_config_index_addr  reg_rwmode=Read/Write  reg_msb=7  reg_lsb=0  reg_mode=Specify via dialog  reg_type=uint(8)  reg_scale=2^0  reg_init=PRACH_regs(InstanceNumber).PRACH_config_index  reg_desc=PRACH_regs(InstanceNumber).PRACH_config_index_string  reg_modal=off  reg_desc0=0  reg_desc1=0  reg_desc2=0  reg_desc3=0  reg_desc4=0  reg_desc5=0  reg_desc6=0  reg_desc7=0  reg_addr=8  SampleTime=-1  version=20090407
  RegField2 : DSPBAModelBus/RegField  reg_name=PRACH_regs(InstanceNumber).PRACH_time_index_addr  reg_rwmode=Read/Write  reg_msb=2  reg_lsb=0  reg_mode=Specify via dialog  reg_type=uint(3)  reg_scale=2^0  reg_init=PRACH_regs(InstanceNumber).PRACH_time_index  reg_desc=PRACH_regs(InstanceNumber).PRACH_time_index_string  reg_modal=off  reg_desc0=0  reg_desc1=0  reg_desc2=0  reg_desc3=0  reg_desc4=0  reg_desc5=0  reg_desc6=0  reg_desc7=0  reg_addr=9  SampleTime=-1  version=20090407
  RegField3 : DSPBAModelBus/RegField  reg_name=PRACH_regs(InstanceNumber).PRACH_NRPRACHSlot_addr  reg_rwmode=Read/Write  reg_msb=0  reg_lsb=0  reg_mode=Specify via dialog  reg_type=uint(1)  reg_scale=2^0  reg_init=PRACH_regs(InstanceNumber).PRACH_NRPRACHSlot  reg_desc=PRACH_regs(InstanceNumber).PRACH_NRPRACHSlot_string  reg_modal=off  reg_desc0=0  reg_desc1=0  reg_desc2=0  reg_desc3=0  reg_desc4=0  reg_desc5=0  reg_desc6=0  reg_desc7=0  reg_addr=10  SampleTime=-1  version=20090407
  RegField4 : DSPBAModelBus/RegField  reg_name=PRACH_regs(InstanceNumber).PRACH_ActivePRACHSlot_addr  reg_rwmode=Read/Write  reg_msb=0  reg_lsb=0  reg_mode=Specify via dialog  reg_type=uint(1)  reg_scale=2^0  reg_init=PRACH_regs(InstanceNumber).PRACH_ActivePRACHSlot  reg_desc=PRACH_regs(InstanceNumber).PRACH_ActivePRACHSlot_string  reg_modal=off  reg_desc0=0  reg_desc1=0  reg_desc2=0  reg_desc3=0  reg_desc4=0  reg_desc5=0  reg_desc6=0  reg_desc7=0  reg_addr=11  SampleTime=-1  version=20090407
  RisingEdgeDetect : Subsystem
  SRlatch_PS : Subsystem  AncestorBlock=DSPBAControl/SRlatch_PS  mask(SetResetLatchPrioritySet){}
      mask help: DSP Builder offers two single-cycle latency latch subsystems for common operations for the valid signal, latching with set and reset. The SRlatch block gives priority to the reset input signal; the SRlatch_PS block gives priority to the set input signal. In both blocks, if set and reset inputs are both zero the current output state is maintained.
      mask Help: helpview(dspba.GetHelp('SRlatch_PS'));
      mask Display:
      | color('w');
      | image('dspba_prim_masked.png');
      | fprintf('SRlatch\nPriority\nSet');
      | port_label('input',1,'s');
      | port_label('input',2,'r');
      | port_label('output',1,'q');
  Select : DSPBAPrim/Select  primtype=select  nInputs=str2num(get_param(gcb,'value'))*2+1  nOutputs=1  omode=Inherit via internal rule  otype=sfix(16)  scale=2^-15  rndmethod=Unbiased  factor=1  satmethod=Symmetric  shift_vec=[0 1 2 -1]  value=1  inPortNames=['d'; '0'; 'a'; '1'; 'b'; '2'; 'c'; '3'; 'd'; '4'; 'e'; '5'; 'f'; '6'; 'g'; '7'; 'h'; '8'; 'i'; '9'; 'j']  outPortNames=[' ']  dspbaimage=dspba_prim_tall.svg  text=fprintf('%s', primtype);  style=Optimised  visibilities=8 + 1024  version=20211007
  StartOfSymbol_LUT : DSPBAPrim/Lut  primtype=lut  nInputs=1  nOutputs=1  omode=Inherit via internal rule  otype=sfix(16)  scale=2^-15  rndmethod=Unbiased  factor=1  satmethod=Symmetric  shift_vec=[0 1 2 -1]  value=ConfigTable(:,13)  inPortNames=[' '; ' ';]  outPortNames=[' ']  dspbaimage=dspba_prim.svg  text=fprintf('LUT');  style=Optimised  visibilities=8 + 1024  floatPrecision=float32_m23  version=20211007
  Sub : DSPBAPrim/Sub  primtype=sub  nInputs=2  nOutputs=1  omode=Specify via dialog  otype=uint(8)  scale=1  rndmethod=Unbiased  factor=1  satmethod=Symmetric  shift_vec=[0 1 2 -1]  value=0  inPortNames=['+'; '-';]  outPortNames=[' ']  dspbaimage=dspba_prim.svg  text=fprintf('-');  style=Optimised  visibilities=8+2^17+2^18  floatRounding=correct  advOptions=[]  version=20211007
  SynthesisInfo : DSPBAPrim/SynthesisInfo  primtype=synthinfo  nInputs=0  nOutputs=0  omode=Inherit via internal rule  otype=sfix(16)  scale=2^-15  rndmethod=Truncate  factor=1  satmethod=Symmetric  shift_vec=[0 1 2 -1]  value=99  inPortNames=[' '; ' ';]  outPortNames=[' ']  dspbaimage=dspba_prim_ctrl.jpg  text=fprintf('Style=%s', style);  style=Scheduled  visibilities=2^15+2^17+2^18+2^19  constraintPair=None  constraintRelation=>  constraintLimit=2  modelRefSign=+  modelRef=''  showSchedule=off  simulationMode=Use Global Value  resetMinimization=Conditional - On for ChannelIn/Out only  version=20220106
  Terminator : Terminator
  Xor : DSPBAPrim/Xor  primtype=xor  nInputs=2  nOutputs=1  omode=Inherit via internal rule  otype=sfix(16)  scale=2^-15  rndmethod=Unbiased  factor=1  satmethod=Symmetric  shift_vec=[0 1 2 -1]  value=0  inPortNames=[' '; ' '; ' '; ' '; ' '; ' '; ' '; ' '; ' '; ' '; ' '; ' '; ' '; ' '; ' '; ' '; ]  outPortNames=[' ']  dspbaimage=dspba_prim.svg  text=fprintf('^');  style=Optimised  visibilities=8+2  version=20211007
  rem : Subsystem
  dout : Outport  VectorParamsAs1DForOutWhenUnconnected=off
  vout : Outport  Port=2  VectorParamsAs1DForOutWhenUnconnected=off
  cout : Outport  Port=3  VectorParamsAs1DForOutWhenUnconnected=off
  CPLen : Outport  Port=4  VectorParamsAs1DForOutWhenUnconnected=off
  FFTSize : Outport  Port=5  VectorParamsAs1DForOutWhenUnconnected=off
  NFFTs : Outport  Port=6  VectorParamsAs1DForOutWhenUnconnected=off
  SOP : Outport  Port=7  VectorParamsAs1DForOutWhenUnconnected=off
  qBWby10 : Outport  Port=8  VectorParamsAs1DForOutWhenUnconnected=off
  TimeReference : Outport  Port=9  VectorParamsAs1DForOutWhenUnconnected=off
  tag scope: X=scoped, Y=scoped
  wires:
  LutY/1 -> [Y], CmpEQ12/2  "Y"
  LutX/1 -> [X]  "X"
  Mux/1 -> ActiveSubF_LUT/1
  ActiveSubF_LUT/1 -> CmpEQ11/2, Display/1
  ChannelI3n/3 -> ConfigValidScope/6, ChannelOu3t/3
  ChannelI3n/4 -> BitCombine/4, CmpEQ11/1
  din/1 -> ChannelI3n/3
  chin/1 -> ChannelI3n/2
  vin/1 -> ChannelI3n/1
  ChannelI3n/2 -> ChannelOu3t/2, ConfigValidScope/5
  ChannelOu3t/3 -> dout/1
  ChannelOu3t/2 -> cout/1
  ChannelOu3t/1 -> vout/1
  ChannelI3n/1 -> ConfigValidScope/2, And2/1
  RegField1/1 -> DisplayConfigIdx/1, DecodeFormat/1(In1), Sub/1
  ChannelI3n/5 -> BitCombine/5, rem/1(SFN)
  rem/1(rem) -> CmpEQ12/1  "remX"
  CmpEQ12/1 -> And1/2  "ActiveSFN"
  And2/1 -> SRlatch_PS/2(r), ConfigValidScope/1, ChannelOu3t/1
  Demux/1 -> Or1/1
  Demux/2 -> Or1/2
  Demux/3 -> Or1/3
  Demux/4 -> Or1/4
  Demux/5 -> Or1/5
  Demux/6 -> Or1/6
  Demux/7 -> Or1/7
  Demux/8 -> Or1/8
  Demux/9 -> Or1/9
  Demux/10 -> Or1/10
  CmpEQ11/1 -> Demux/1
  Sub/1 -> LutX/1, PRACHSymDuration_LUT/1, PrachOccPerSlotMinus1/1, NrPRrachSlot_LUT/1, StartOfSymbol_LUT/1, LutY/1, DisplayConfigIdx1/1, Mux/1, Mux/2, Mux/3, Mux/4, Mux/5, Mux/6, Mux/7, Mux/8, Mux/9, Mux/10
  Const3/1 -> Sub/2
  SubFN/1 -> ChannelI3n/4
  SFN/1 -> ChannelI3n/5
  CPLenDecode/1(CPLen) -> Add2/1, Display3/1
  ChannelOu3t/4 -> CPLen/1
  ChannelOu3t/5 -> FFTSize/1
  SCSby15/1 -> ChannelI3n/6
  BWby10/1 -> ChannelI3n/7
  ChannelI3n/6 -> FFTSizeDecode/1(SCSby15)
  ChannelI3n/7 -> FFTSizeDecode/2(BW/10), ChannelOu3t/8
  FFTSizeDecode/2(k) -> CPLenDecode/1(k), DisplayK/1
  FFTSizeDecode/3(mu) -> CPLenDecode/2(mu), DisplayMu/1
  [X] -> DisplayX/1
  [Y] -> DisplayY/1
  NumberOfFFTDecode/1(NFFTs) -> ChannelOu3t/6, DisplayNFFTs/1, BitCombine/2
  ChannelOu3t/6 -> NFFTs/1
  And1/1 -> RisingEdgeDetect/1(SigIn), And2/2, ConfigValidScope/3
  Or1/1 -> And1/1  "ActiveSubFN"
  ChannelOu3t/7 -> SOP/1
  RisingEdgeDetect/1(PosEdge) -> ConfigValidScope/7, SRlatch_PS/1(s)
  FFTSizeDecode/1(FFTSize) -> DisplayLog2FFTSize/1, ChannelOu3t/5
  FFTSizeDecode/4(FFTPoints_Plus_OFDMCP) -> Mult1/1, DisplayStartOfPrach3/1, DisplayOfdmCP/1
  RegField2/1 -> DisplayTimeIndex/1, CmpEQ/2, Mult/2
  PRACHSymDuration_LUT/1 -> DisplayPrachSymDuration/1, Mult/1
  Mult/1 -> DisplayTimeIndexXSymDuration/1, Add/2
  StartOfSymbol_LUT/1 -> DisplayStartOfSymbol/1, BitCombine/1, Add/1
  Add/1 -> Mult1/2, DisplayTimeIndexXSymDurationPlusStartOfSym/1
  Mult1/1 -> DisplayStartOfPrach2/1, Add1/2
  FFTSizeDecode/5(SymPerSFby2timesNfft) -> Select/3
  RegField3/1 -> Xor/1
  RegField4/1 -> Xor/2
  Select/1 -> DisplayStartOfPrach1/1, Add1/1
  Xor/1 -> DisplayAxBxSel/1, BitCombine/3, Select/2
  Const1/1 -> Select/1
  Add1/1 -> Add2/2, DisplayStartOfPrach/1
  Add2/1 -> ChannelOu3t/4
  ChannelOu3t/8 -> qBWby10/1
  SRlatch_PS/1(q) -> ChannelOu3t/7, ConfigValidScope/4
  CmpEQ/1 -> CPLenDecode/3(time_index)
  NrPRrachSlot_LUT/1 -> Terminator/1
  PrachOccPerSlotMinus1/1 -> CmpEQ/1, DisplayPrachOccPerSlotMinus1/1
  BitCombine/1 -> ChannelOu3t/9
  ChannelOu3t/9 -> TimeReference/1
